simulink model "ardupilotsailboat"  (R2022b)
settings: Solver=VariableStepAuto  StartTime=0.0  StopTime=250  RelTol=1e-3
values from neighbouring files (symbols this model uses):
  Ixx = 1/120 * pi * rho * L * B * T * (4*T^2 + B^2)    (= 0.835683076278)    [parameterCalculations.m]
  m = 2    [parameterCalculations.m]
  m11 = m*k11    [parameterCalculations.m]
  m22 = m*k22    [parameterCalculations.m]
  Yv = Yv * (u^2)/(U^2)    (= -23.3298597446)    [parameterCalculations.m]
undefined symbols (not defined in the file or in its folder): Waypoints
libraries: cstblocks x6, simulink x1, vrlib x1
(part 1 of 2)
settings Model: Creator=ruben  LastModifiedBy=ruben
settings SolverCC: MaxConsecutiveZCs=10  MaxConsecutiveMinStep=9  ZeroCrossControl=DisableAll  ZeroCrossAlgorithm=Adaptive  SolverResetMethod=Robust
settings DebuggingCC: SignalInfNanChecking=warning  AlgebraicLoopMsg=error  ArtificialAlgebraicLoopMsg=error  BlockPriorityViolationMsg=error  MinStepSizeMsg=error  MaskedZcDiagnostic=error  IgnoredZcDiagnostic=none  MultiTaskCondExecSysMsg=warning  MultiTaskRateTransMsg=warning  CheckMatrixSingularityMsg=error  StateNameClashWarn=warning

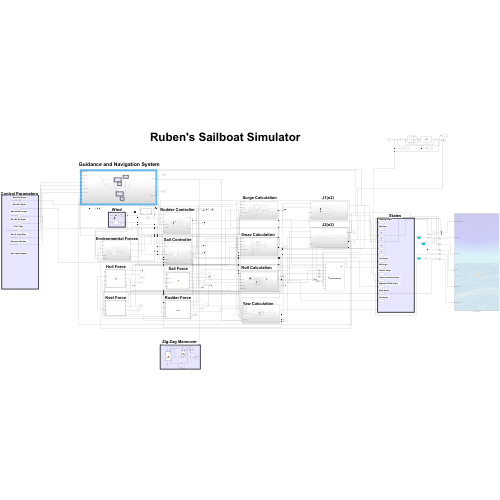
[thumbnail: Simulink's stored preview of the top-level diagram]
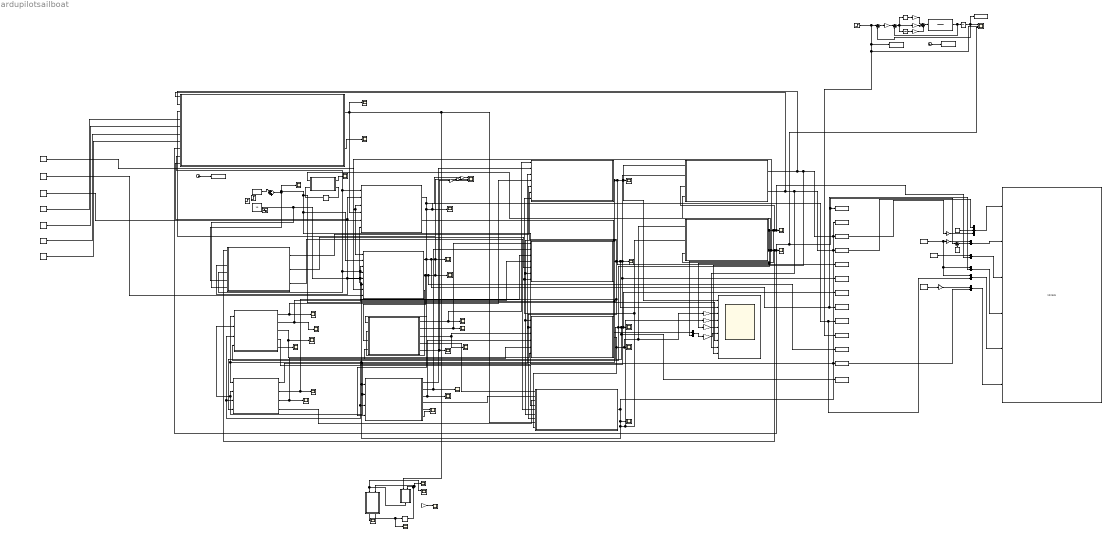
== system ardupilotsailboat ==
  note: Sail Force
  note: Ruben's Sailboat Simulator
  note: States
  note: x
  note: y
  note: Yaw Rate
  note: Heading Angle
  note: u
  note: v
  note: Roll Angle
  note: Sail Angle
  note: Rudder Angle
  note: Desired Heading Angle
  note: Apparent Wind Angle
  note: Wind Angle
  note: Roll Angle
  note: Guidance and Navigation System
  note: Environmental Forces
  note: Surge Calculation
  note: Sway Calculation
  note: Roll Calculation
  note: Yaw Calculation
  note: Wind
  note: Rudder Force
  note: Keel Force
  note: Hull Force
  note: Sail Controller
  note: Rudder Controller
  note: Zig-Zag Maneuver
  note: Control Parameters
  note: Max Sail Angle
  note: Min Sail Angle
  note: Sail No Go Angle
  note: Sail X-Track Max
  note: Sail Loiter Raduis
  note: Waypoint Radius
  note: Tack Type
  note: Max Rudder Angle
  note: J1(n2)
  note: J2(n2)
  Bus Creator : BusCreator  Inputs=2
  Clock : Clock
  Clock2 : Clock
  Cross-Track Distance(m) : Constant  Value=7.5
  Delay1 : Delay  DelayLength=1  SampleTime=0.01
  Delay2 : Delay  DelayLength=1  SampleTime=0.01
  Derivative : Derivative
  Gain : Gain  Gain=0.0225
  Gain{1..8} (8 alike) : Gain  Gain=180/pi
  Gain10 : Gain
  Gain11 : Gain  Gain=0.99
  Gain9 : Gain  Gain=2.66
  Integrator : Integrator
  Integrator1 : Integrator
  MATLAB Function1 : MATLAB Function  TreatAsAtomicUnit=on
  MATLAB Function3 : MATLAB Function  TreatAsAtomicUnit=on
  MATLAB Function4 : MATLAB Function  TreatAsAtomicUnit=on
  MATLAB Function5 : MATLAB Function  TreatAsAtomicUnit=on
  MATLAB Function6 : MATLAB Function  TreatAsAtomicUnit=on
  MATLAB Function7 : MATLAB Function  TreatAsAtomicUnit=on
  MATLAB Function8 : MATLAB Function  TreatAsAtomicUnit=on
  Mux1 : Mux  Inputs=3
  Mux{2,4..7} (5 alike) : Mux  Inputs=2
  Radius of Acceptance(m) : Constant  Value=5
  Roll Axis of Rotation : Constant  Value=[ -1 0 0 ]
  Scope{,1..14,16..17,33,35,37..38,40,42} (23 alike) : Scope
  Scope15 : Scope  NumInputPorts=3
  Scope18 : Scope  NumInputPorts=3
  Scope36 : Scope  NumInputPorts=9
  Scope41 : Scope  NumInputPorts=2
  Sine Wave : Sin  Amplitude=0.1  Frequency=0.1  SampleTime=0
  Step : Step  Time=19  After=0.25  SampleTime=0
  Step1 : Step  Time=40  After=0.5  SampleTime=0
  Step2 : Step  After=0.1  SampleTime=0
  Subsystem1 : Subsystem
  Subsystem10 : Subsystem
  Subsystem2 : Subsystem
  Subsystem3 : Subsystem
  Subsystem4 : Subsystem
  Subsystem5 : Subsystem
  Subsystem6 : Subsystem
  Subsystem7 : Subsystem
  Subsystem8 : Subsystem
  Subsystem9 : Subsystem
  Sum : Sum  Inputs=|++-+
  Sum1 : Sum  Inputs=|+-  SaturateOnIntegerOverflow=on
  Sum2 : Sum  Inputs=|+-
  Sum3 : Sum  Inputs=|+++
  Sum4 : Sum  Inputs=|+-
  "Tack Type (1:Direct, 2:Indirect 3:Zone)" : Constant
  To Workspace : ToWorkspace  VariableName=yawrate  SaveFormat=Timeseries  SampleTime=-1
  To Workspace1 : ToWorkspace  VariableName=yaw  SaveFormat=Timeseries  SampleTime=-1
  To Workspace10 : ToWorkspace  VariableName=psid  SaveFormat=Timeseries  SampleTime=-1
  To Workspace11 : ToWorkspace  VariableName=awa  SaveFormat=Timeseries  SampleTime=-1
  To Workspace12 : ToWorkspace  VariableName=wind  SaveFormat=Timeseries  SampleTime=-1
  To Workspace13 : ToWorkspace  VariableName=roll  SaveFormat=Timeseries  SampleTime=-1
  To Workspace14 : ToWorkspace  VariableName=time1  SaveFormat=Timeseries  SampleTime=-1
  To Workspace15 : ToWorkspace  VariableName=time  SaveFormat=Timeseries  SampleTime=-1
  To Workspace16 : ToWorkspace  VariableName=step  SaveFormat=Timeseries  SampleTime=-1
  To Workspace2 : ToWorkspace  VariableName=simout  SaveFormat=Timeseries  SampleTime=-1
  To Workspace3 : ToWorkspace  VariableName=x  SaveFormat=Timeseries  SampleTime=-1
  To Workspace4 : ToWorkspace  VariableName=y  SaveFormat=Timeseries  SampleTime=-1
  To Workspace5 : ToWorkspace  VariableName=u  SaveFormat=Timeseries  SampleTime=-1
  To Workspace6 : ToWorkspace  VariableName=v  SaveFormat=Timeseries  SampleTime=-1
  To Workspace7 : ToWorkspace  VariableName=phi  SaveFormat=Timeseries  SampleTime=-1
  To Workspace8 : ToWorkspace  VariableName=delta_s  SaveFormat=Timeseries  SampleTime=-1
  To Workspace9 : ToWorkspace  VariableName=delta_r  SaveFormat=Timeseries  SampleTime=-1
  Transfer Fcn : TransferFcn  Numerator=[2.5]  Denominator=[0.4 1 ]
  VR Sailing Yacht Animation : vrlib/VR Sink  InstantiateOnLoad=on  SampleTime=0.05  ViewEnable=on  RemoteChange=off  RemoteView=off  FieldsWritten=Hull_EarthFixed.translation.3.1.1.double#Rot_Yaw.rotation.4.1.1.double#Rot_Roll.rotation.4.1.1.double#Sail.rotation.4.1.1.double#Rudder.rotation.4.1.1.double#Wind_Arrow.rotation.4.1.1.double  WorldFileName=SailingYachtAnimation.wrl  WorldDescription=Sailing Yacht VR animation  AutoView=on  VideoDimensions=[]  AllowVariableSize=off  FigureProperties="{'Position', 'Name', 'Viewpoint', 'CameraBound', 'CameraDirection', 'CameraPosition', 'CameraUpVector', 'ZoomFactor', 'Antialiasing', 'Headlight', 'Lighting', 'NavPanel', 'Sound', 'StatusBar', 'Stereo3D', 'Stereo3DCameraOffset', 'Stereo3DHIT', 'ToolBar', 'Textures', 'Transparency', 'Triad', 'Wireframe', 'NavZones', 'NavMode', 'NavSpeed', 'CaptureFileFormat', 'CaptureFileName', 'Record2DCompressMethod', 'Record2DCompressQuality', 'Record2D', 'Record2DFileName', 'Record2DFPS'; [9.6200000000000000e+02   8.4000000000000000e+01   9.5800000000000000e+02   3.8020000000000005e+02], 'Sailing Yacht VR animation', 'North', 'on', [0.0000000000000000e+00   0.0000000000000000e+00  -1.0000000000000000e+00], [0.0000000000000000e+00   0.0000000000000000e+00   2.5000000000000000e+01], [0.0000000000000000e+00   1.0000000000000000e+00   0.0000000000000000e+00], [1.0000000000000000e+00], 'off', 'on', 'on', 'halfbar', 'on', 'on', 'off', [1.0000000149011612e-01], [0.0000000000000000e+00], 'on', 'on', 'on', 'none', 'off', 'off', 'fly', 'veryfast', 'tif', '%f_anim_%n.tif', 'auto', [7.5000000000000000e+01], 'off', '%f_anim_%n.avi', 'auto'}"
  Yaw Axis of Rotation : Constant  Value=[ 0 1 0 ]
  Yaw Axis of Rotation1 : Constant  Value=[ 0 1 0 ]
  apparent wind : Scope
  max rudder angle(Rad) : Constant  Value=pi/6
  max sail angle(Rad) : Constant  Value=pi/3
  min sail angle(Rad) : Constant  Value=-pi/3
  rudder and psi1 : Scope  NumInputPorts=2
  rudder angle5 : Scope
  rudder angle6 : Scope
  rudder angle7 : Scope  NumInputPorts=3
  rudder angle8 : Scope
  rudder_angle1 : Scope
  sail angle : Scope
  sail no go angle(Degrees) : Constant  Value=45
  wind direction : Constant  Value=pi/2
  wind velocity : Constant  Value=10
  z : Constant  Value=0
  z - y1 : Gain  Gain=-1
  z - y2 : Gain  Gain=-1
  z - y3 : Gain  Gain=-1
  z1 : Constant  Value=pi/2
  wires:
  Subsystem1/2(heading (degrees)) -> Scope33/1
  MATLAB Function3/2(Ys) -> Scope1/1, Subsystem4/1(sail force (Ys))
  MATLAB Function3/3(Ks) -> Scope14/1, Subsystem5/3(sail force (Ks))
  MATLAB Function3/4(Ns) -> Subsystem6/1(sail force (Ns))
  MATLAB Function4/1(Xr) -> Subsystem2/2(rudder force (Xr))
  MATLAB Function4/2(Yr) -> Scope2/1, Subsystem4/2(rudder force (Yr))
  MATLAB Function4/3(Kr) -> Scope13/1, Subsystem5/4(hull force(Kh))
  MATLAB Function4/4(Nr) -> Subsystem6/2(rudder force (Nr))
  MATLAB Function5/1(Xk) -> Subsystem2/3(keel force (Xk))
  MATLAB Function5/2(Yk) -> Scope3/1, Subsystem4/3(keel force (Yk))
  MATLAB Function5/3(Kk) -> Scope12/1, Subsystem5/5(keel force (Kk))
  MATLAB Function5/4(Nk) -> Subsystem6/3(keel force (Nk))
  MATLAB Function6/1(Xh) -> Scope5/1, Subsystem2/4(hull force (Xh))
  MATLAB Function6/3(Kh) -> Scope11/1, Subsystem5/6(rudder force (Kr))
  MATLAB Function6/4(Nh) -> Subsystem6/4(hull force (Nh))
  Subsystem4/1(v) -> Scope36/2, Scope8/1, Subsystem9/2(v), To Workspace6/1, MATLAB Function6/3(v), MATLAB Function5/3(v), MATLAB Function4/3(v), Subsystem2/6(v), Subsystem6/7(v), Subsystem5/2(v), Subsystem8/2(v), Subsystem1/10(v), Subsystem3/3(v), Subsystem7/4(v)
  Subsystem3/1(Xe) -> Subsystem2/5(environmental force (Xe))
  Subsystem3/2(Ye) -> Subsystem4/5(environmental force (Ye))
  Subsystem3/3(Ne) -> Subsystem6/5(environmental force (Ne))
  Subsystem2/1(u) -> MATLAB Function5/2(u), MATLAB Function6/2(u), MATLAB Function4/2(u), Subsystem1/9(u), Subsystem8/1(u), Subsystem3/4(u), Subsystem7/3(u), Subsystem6/6(u), Subsystem5/1(u), Subsystem4/6(u), To Workspace5/1, Scope36/1, Subsystem9/1(u), Scope35/1
  Subsystem6/1(r) -> Subsystem8/6(r), Subsystem7/6(r), MATLAB Function5/1(r), MATLAB Function6/1(r), MATLAB Function4/1(r), Gain4/1, Subsystem10/2(r), Subsystem2/7(r), Subsystem4/7(r), Scope40/1, To Workspace/1
  Subsystem5/1(p) -> Subsystem6/9(p), Subsystem10/1(p), Gain5/1, Scope38/1
  Subsystem10/1(Phi) -> Gain3/1, MATLAB Function5/4(phi), MATLAB Function6/4(phi), To Workspace13/1, MATLAB Function3/4(phi), To Workspace7/1, Scope37/1, Subsystem10/3(phi), Subsystem9/3(phi), Mux6/2, Scope9/1
  Clock2/1 -> To Workspace14/1
  MATLAB Function7/2(nextState) -> rudder angle5/1, Delay1/1
  Delay1/1 -> rudder angle8/1, MATLAB Function8/2(state), MATLAB Function7/2(currentState)
  MATLAB Function7/1(y) -> rudder angle6/1
  MATLAB Function8/1(y) -> MATLAB Function7/1(r), rudder angle7/1
  Gain2/1 -> rudder and psi1/1
  wind velocity/1 -> Subsystem3/6(wind Velocity), Subsystem7/5(wind velocity)
  Subsystem7/1(sail angle) -> MATLAB Function3/1(delta_s), Gain7/1, sail angle/1, Mux5/2, To Workspace8/1
  Subsystem7/2(alpha_aw) -> To Workspace11/1, Subsystem1/3(wind Direction), apparent wind/1, MATLAB Function3/3(apparent_wind_angle)
  Subsystem7/3(V_aw) -> MATLAB Function3/2(apparent_velocity)
  Subsystem8/1(rudder angle) -> Gain8/1, To Workspace9/1, Mux7/2, rudder_angle1/1, MATLAB Function4/4("delta_r ")
  MATLAB Function4/5(delta_r) -> Scope41/1
  MATLAB Function4/6(alpha_a) -> Scope41/2
  MATLAB Function6/2(Yh) -> Subsystem4/4(hull force (Yh)), Scope4/1
  max sail angle(Rad)/1 -> Subsystem7/7(max sail angle)
  min sail angle(Rad)/1 -> Subsystem7/8(min sail angle)
  max rudder angle(Rad)/1 -> Subsystem8/5(max rudder angle)
  sail no go angle(Degrees)/1 -> Subsystem1/4(no go Angle)
  "Tack Type (1:Direct, 2:Indirect 3:Zone)"/1 -> Subsystem1/5(tack Type)
  Cross-Track Distance(m)/1 -> Subsystem1/6(Cross-Track Distance)
  Radius of Acceptance(m)/1 -> Subsystem1/7(radius of acceptance)
  wind direction/1 -> Sum/1
  MATLAB Function6/5(Frh) -> Scope6/1
  MATLAB Function3/1(Xs) -> Subsystem2/1(sail force (Xs)), Scope7/1
  Subsystem9/2(y) -> Subsystem1/1(x position of Sailboat), Scope36/8, Mux1/1, To Workspace3/1
  Subsystem8/2(rudder angle1) -> Bus Creator/1
  Subsystem10/2(Psi) -> MATLAB Function1/1(psi), Bus Creator/2, Subsystem9/4(psi), Subsystem7/1(psi), Subsystem8/3(psi), Subsystem3/1(psi), Scope18/3, Sum1/1, To Workspace1/1, Subsystem1/8(psi), Scope10/1
  Bus Creator/1 -> Gain1/1
  z1/1 -> Sum1/2
  z - y1/1 -> Mux4/1
  Yaw Axis of Rotation/1 -> Mux5/1, Mux7/1, z - y1/1
  z/1 -> Mux1/2
  z - y3/1 -> Mux2/1
  Mux2/1 -> VR Sailing Yacht Animation/6
  Sum1/1 -> Mux4/2
  Yaw Axis of Rotation1/1 -> z - y3/1
  z - y2/1 -> Mux1/3
  Roll Axis of Rotation/1 -> Mux6/1
  Mux1/1 -> VR Sailing Yacht Animation/1
  Mux4/1 -> VR Sailing Yacht Animation/2
  Mux6/1 -> VR Sailing Yacht Animation/3
  Mux5/1 -> VR Sailing Yacht Animation/4
  Mux7/1 -> VR Sailing Yacht Animation/5
  Subsystem9/1(x) -> Subsystem1/2(y position of Sailboat), Scope36/9, z - y2/1, To Workspace4/1
  MATLAB Function3/5(awa) -> Gain6/1, Scope42/1
  Gain3/1 -> Scope36/5
  Gain1/1 -> Scope36/6
  Gain4/1 -> Scope36/4
  Gain5/1 -> Scope36/3
  Gain6/1 -> Scope15/3
  Gain7/1 -> Scope15/2
  Gain8/1 -> Scope15/1
  MATLAB Function1/2(nextState) -> Delay2/1
  Delay2/1 -> MATLAB Function1/2(currentState)
  MATLAB Function1/1(y) -> Scope16/1
  Sum/1 -> Scope17/1, Scope36/7, Mux2/2, To Workspace12/1, Subsystem7/2(wind direction), Subsystem3/5(wind Direction)
  Clock/1 -> To Workspace15/1
  Integrator/1 -> Gain10/1
  Derivative/1 -> Gain/1
  Gain9/1 -> Sum3/2
  Transfer Fcn/1 -> Sum2/2, Integrator1/1
  Sum2/1 -> Derivative/1, Gain9/1, Integrator/1
  Gain/1 -> Sum3/1
  Sum3/1 -> Transfer Fcn/1
  Gain10/1 -> Sum3/3
  Step2/1 -> Sum4/1, Scope18/2, To Workspace10/1, To Workspace16/1
  Integrator1/1 -> Sum4/2, Scope18/1, To Workspace2/1
  Sum4/1 -> Gain11/1
  Gain11/1 -> Sum2/1
  Subsystem1/1(heading (rad)) -> Scope/1, Subsystem8/4(desired heading), Subsystem6/8(desired heading), MATLAB Function8/1(psi)

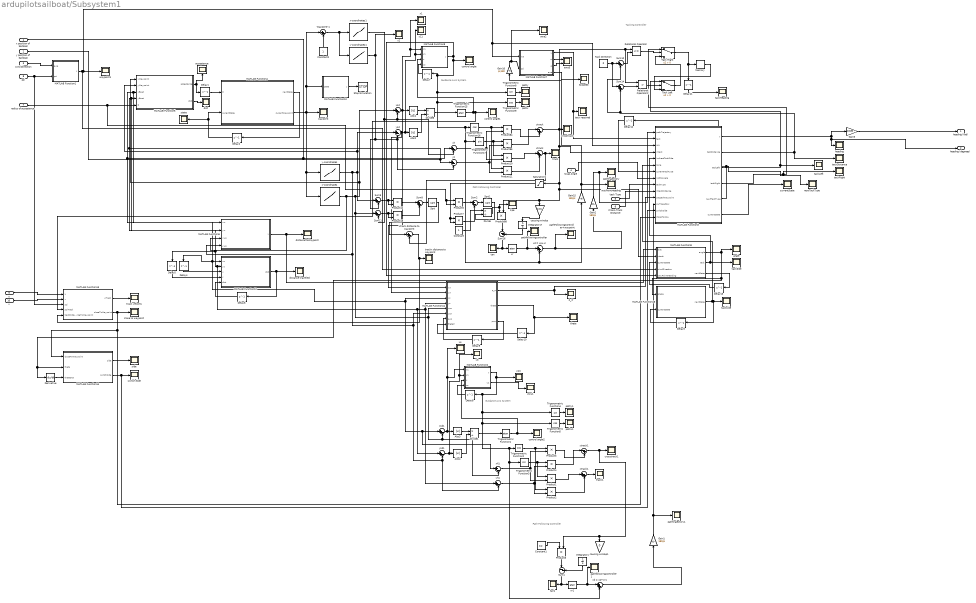
== system ardupilotsailboat/Subsystem1 ==
  note: Guidance Axis System
  note: Tacking Controller
  note: Path Following Controller
  note: Guidance Axis System
  note: Path Following Controller
  x position of Sailboat : Inport
  y position of Sailboat : Inport  Port=2
  wind Direction : Inport  Port=3
  no go Angle : Inport  Port=4
  tack Type : Inport  Port=5
  Cross-Track Distance : Inport  Port=6
  radius of acceptance : Inport  Port=7
  psi : Inport  Port=8
  u : Inport  Port=9
  v : Inport  Port=10
  Abs{1..4} (4 alike) : Abs  SaturateOnIntegerOverflow=off
  Constant : Constant
  Constant1 : Constant  Value=0.2
  Constant2 : Constant
  Delay{1..2,4..12} (11 alike) : Delay  DelayLength=1
  Delay13 : Delay  DelayLength=1  SampleTime=2
  Delay3 : Delay  DelayLength=1  SampleTime=2
  Derivative : Derivative
  Divide : Product  Inputs=*/
  Divide1 : Product  Inputs=*/
  Divide6 : Product  Inputs=*/
  Gain1 : Gain  Gain=180/pi
  Gain10 : Gain  Gain=pi/180
  Gain15 : Gain  Gain=180/pi
  Gain2 : Gain  Gain=180/pi
  Gain3 : Gain  Gain=pi/180
  Integrator1 : Integrator  LimitOutput=on  UpperSaturationLimit=10  LowerSaturationLimit=-10
  Integrator17 : Integrator  LimitOutput=on  UpperSaturationLimit=pi/10  LowerSaturationLimit=-pi/10
  Kpe : Scope
  MATLAB Function1 : MATLAB Function  TreatAsAtomicUnit=on
  MATLAB Function10 : MATLAB Function  TreatAsAtomicUnit=on
  MATLAB Function11 : MATLAB Function  TreatAsAtomicUnit=on
  MATLAB Function12 : MATLAB Function  TreatAsAtomicUnit=on
  MATLAB Function13 : MATLAB Function  TreatAsAtomicUnit=on
  MATLAB Function14 : MATLAB Function  TreatAsAtomicUnit=on
  MATLAB Function18 : MATLAB Function  TreatAsAtomicUnit=on
  MATLAB Function2 : MATLAB Function  TreatAsAtomicUnit=on
  MATLAB Function3 : MATLAB Function  TreatAsAtomicUnit=on
  MATLAB Function4 : MATLAB Function  TreatAsAtomicUnit=on
  MATLAB Function5 : MATLAB Function  TreatAsAtomicUnit=on
  MATLAB Function6 : MATLAB Function  TreatAsAtomicUnit=on
  MATLAB Function7 : MATLAB Function  TreatAsAtomicUnit=on
  MATLAB Function8 : MATLAB Function  TreatAsAtomicUnit=on
  MATLAB Function9 : MATLAB Function  TreatAsAtomicUnit=on
  Memory : Memory
  Product{1..7,10..13,84..85,88} (14 alike) : Product
  Relational Operator : RelationalOperator  Operator=<=  OutDataTypeStr=boolean  RndMeth=Simplest  InputSameDT=off
  Relational Operator1 : RelationalOperator  Operator=>  OutDataTypeStr=boolean  RndMeth=Simplest  InputSameDT=off
  Saturation1 : Saturate  UpperLimit=4.9  LowerLimit=-4.9
  Scope33 : Scope
  Sqrt : Sqrt
  Sqrt1 : Sqrt
  Stop Simulation : Stop
  Sum1 : Sum  Inputs=|--
  Sum{2,9..11} (4 alike) : Sum  Inputs=|+-
  Sum14 : Sum  Inputs=|++
  Sum16 : Sum  Inputs=|--
  Sum8 : Sum  Inputs=|++
  Tack Direction : Constant  Value=0
  Tack Left : Switch  Criteria=u2 > Threshold  SaturateOnIntegerOverflow=off  InputSameDT=off
  Tack Right : Switch  Criteria=u2 > Threshold  SaturateOnIntegerOverflow=off  InputSameDT=off
  Trigonometric Function1 : Trigonometry  Operator=atan
  Trigonometric Function15 : Trigonometry  Operator=atan
  Trigonometric Function{2,5,9,16} (4 alike) : Trigonometry  Operator=cos
  Trigonometric Function{3..4,8,17} (4 alike) : Trigonometry
  Waypoint-1 : Sum  Inputs=|+-
  acceptance : Scope
  angle : Scope
  awa2 : Scope
  awa3 : Scope  NumInputPorts=2
  causing windup : Gain  Gain=0.01
  causing windup1 : Gain  Gain=0
  close to waypoint : Scope
  control angle : Scope
  control angle1 : Scope
  control angle2 : Scope
  crosstrack : Scope
  crosstrack1 : Scope
  currentState : Scope
  dist : Scope
  distance travelled : Scope
  distanceToWaypoint : Scope
  heading : Scope
  nextTackType : Scope
  p_w : Scope
  "pathFollowingController+waypoint " : Scope
  pathfollowingcontroller : Scope
  pathfollowingcontroller1 : Scope
  pathtrajectory : Scope
  pathtrajectory1 : Scope
  pathx : Scope
  pathx1 : Scope
  pathy : Scope
  pathy1 : Scope
  pwu1 : Scope
  side : Scope
  state : Scope
  switch Side : Scope
  tack required : Scope
  tackDistance : Scope
  tackHeading : Scope
  tackLeft : Scope
  tackRight : Scope
  tackSide : Scope
  tackside : Scope
  tan : Scope
  tan1 : Scope
  theta : Scope
  track : Scope
  track velocity : Scope
  track1 : Scope
  trackx distance to waypoint : Scope
  wayPointHeading : Scope
  waypoint : Scope
  waypoint1 : Scope
  x-coordinates : Lookup_n-D  NumberOfTableDimensions=1  BreakpointsForDimension1=Waypoints.number  Table=Waypoints.x  InterpMethod=Cubic spline  ExtrapMethod=Cubic spline  InternalRulePriority=Speed  RndMeth=Simplest
  x-coordinates1 : Lookup_n-D  NumberOfTableDimensions=1  BreakpointsForDimension1=Waypoints.number  Table=Waypoints.x  InterpMethod=Cubic spline  ExtrapMethod=Cubic spline  InternalRulePriority=Speed  RndMeth=Simplest
  x1 : Scope
  x2 : Scope
  x4 : Scope
  xd = xp+xr : Sum  Inputs=|++
  xd = xp+xr1 : Sum  Inputs=|++
  xh : Sum  Inputs=|+-
  xh1 : Sum  Inputs=|+-
  xr : Trigonometry  Operator=atan
  xr1 : Trigonometry  Operator=atan
  xsd : Sum  Inputs=|+-
  xsd1 : Sum  Inputs=|+-
  xtrack : Sum  Inputs=|++
  xtrack distance to waypoint : Sum  Inputs=|+-
  xtrack1 : Sum  Inputs=|++
  y-coordinates : Lookup_n-D  NumberOfTableDimensions=1  BreakpointsForDimension1=Waypoints.number  Table=Waypoints.y  InterpMethod=Cubic spline  ExtrapMethod=Cubic spline  InternalRulePriority=Speed  RndMeth=Simplest
  y-coordinates1 : Lookup_n-D  NumberOfTableDimensions=1  BreakpointsForDimension1=Waypoints.number  Table=Waypoints.y  InterpMethod=Cubic spline  ExtrapMethod=Cubic spline  InternalRulePriority=Speed  RndMeth=Simplest
  y11 : Scope
  y3 : Scope
  yh : Sum  Inputs=|+-
  yh1 : Sum  Inputs=|+-
  ypw : Scope
  ysd : Sum  Inputs=|+-
  ysd1 : Sum  Inputs=|+-
  ytrack : Sum  Inputs=|-+
  ytrack1 : Sum  Inputs=|-+
  heading (rad) : Outport
  heading (degrees) : Outport  Port=2
  wires:
  MATLAB Function11/2(theta) -> Delay10/1, theta/1
  MATLAB Function7/3(p) -> awa3/2
  Delay2/1 -> MATLAB Function4/2(currentState), state/1
  Trigonometric Function17/1 -> Product10/1, Product85/1
  MATLAB Function3/6(currentState) -> currentState/1
  MATLAB Function3/1(y) -> Gain3/1, heading (degrees)/1, heading/1
  Gain2/1 -> MATLAB Function3/1(pathTrajectory), pathtrajectory/1
  Delay12/1 -> MATLAB Function3/7(currentTackType)
  MATLAB Function4/2(currentWaypoint) -> MATLAB Function10/1(state), Waypoint-1/1, waypoint/1, x-coordinates/1, y-coordinates/1
  yh/1 -> Product85/2, Product11/2
  MATLAB Function7/2(w) -> awa3/1
  Sum14/1 -> Relational Operator1/2
  ytrack/1 -> Saturation1/1, Product88/2, causing windup/1, MATLAB Function9/2(xtrack), MATLAB Function3/4(xtrack), crosstrack/1, Relational Operator1/1, Relational Operator/1
  Product85/1 -> ytrack/1
  Delay11/1 -> tackHeading/1
  MATLAB Function3/2(tackDistance) -> Sum10/2, Sum14/2, tackDistance/1
  Integrator17/1 -> Sum16/2
  Abs1/1 -> Divide6/1
  Trigonometric Function16/1 -> Product11/1, Product84/1
  Delay7/1 -> MATLAB Function8/4(us)
  MATLAB Function18/1(nextState) -> tackside/1, Delay3/1, MATLAB Function3/6(zone)
  xd = xp+xr/1 -> "pathFollowingController+waypoint "/1, Gain2/1
  Gain10/1 -> MATLAB Function7/2(psi), awa2/1
  MATLAB Function3/5(nextTackType) -> Delay12/1, nextTackType/1
  Delay13/1 -> MATLAB Function9/3(currentState)
  Waypoint-1/1 -> x-coordinates1/1, y-coordinates1/1
  Delay3/1 -> MATLAB Function18/2(currentState)
  xsd/1 -> MATLAB Function11/1(xw), MATLAB Function8/1(x1), x1/1, Abs1/1
  Constant2/1 -> Waypoint-1/2
  MATLAB Function8/1(y) -> Trigonometric Function8/1, Trigonometric Function9/1, Trigonometric Function17/1, xd = xp+xr/2, Gain15/1, Trigonometric Function16/1, Delay7/1, control angle/1, MATLAB Function9/5(wayPointHeading)
  xh/1 -> Product84/2, Product10/2
  Delay1/1 -> MATLAB Function4/1(R)
  MATLAB Function9/3(nextState) -> Delay13/1
  Product84/1 -> ytrack/2
  y-coordinates1/1 -> yh/2, ysd/2, Sum9/2, x2/1
  Trigonometric Function15/1 -> MATLAB Function13/4(psiTrack), control angle1/1, MATLAB Function8/3(u)
  ysd/1 -> y11/1, MATLAB Function8/2(y1), Abs2/1, MATLAB Function11/2(yw)
  x-coordinates1/1 -> Sum11/2, xh/2, xsd/2
  Sum16/1 -> xr/1, tan/1
  Product13/1 -> Sum8/2
  Gain15/1 -> Gain10/1, wayPointHeading/1
  MATLAB Function6/1(y) -> MATLAB Function9/1(dist), distanceToWaypoint/1
  Delay5/1 -> MATLAB Function12/4(y)
  MATLAB Function9/1(angle) -> angle/1, Derivative/1, MATLAB Function14/2(theta), MATLAB Function18/1(angle)
  Product88/1 -> Sum16/1
  Relational Operator1/1 -> Tack Left/2
  MATLAB Function3/3(tackLeft) -> Tack Left/1, tackLeft/1
  Tack Right/1 -> Memory/1, Delay11/1
  xtrack distance to waypoint/1 -> MATLAB Function13/5(trackDistanceToWaypoint), trackx distance to waypoint/1
  Memory/1 -> Tack Left/3
  Product11/1 -> xtrack/2
  Trigonometric Function8/1 -> pathy/1
  MATLAB Function7/1(y) -> MATLAB Function3/2(tack), tack required/1
  Delay4/1 -> MATLAB Function12/3(x)
  causing windup/1 -> Integrator17/1
  Tack Left/1 -> Tack Right/3
  MATLAB Function10/1(y) -> Stop Simulation/1
  Sum8/1 -> Sqrt/1
  Sum11/1 -> Product13/2, Product13/1
  Tack Direction/1 -> Sum14/1, Sum10/1
  Sum9/1 -> Product12/1, Product12/2
  Delay6/1 -> MATLAB Function12/5("dist ")
  MATLAB Function5/1(acceptance) -> Delay1/1, acceptance/1
  MATLAB Function12/1(dist) -> distance travelled/1, Delay6/1
  Relational Operator/1 -> Tack Right/2
  Sum10/1 -> Relational Operator/2
  xtrack/1 -> xtrack distance to waypoint/2, track/1
  Abs2/1 -> Divide6/2
  MATLAB Function4/1(nextState) -> Delay2/1
  Sqrt/1 -> xtrack distance to waypoint/1
  MATLAB Function11/1(p_w) -> p_w/1, MATLAB Function3/11(passedWaypoint)
  Product10/1 -> xtrack/1
  xr/1 -> xd = xp+xr/1, pathfollowingcontroller/1
  MATLAB Function3/4(tackRight) -> tackRight/1, Tack Right/1
  Product12/1 -> Sum8/1
  Trigonometric Function9/1 -> pathx/1
  MATLAB Function7/4(awa) -> Scope33/1
  no go Angle/1 -> MATLAB Function3/8(noGoAngle)
  tack Type/1 -> MATLAB Function3/9(tackType)
  Cross-Track Distance/1 -> MATLAB Function3/10(XtrackDistance)
  radius of acceptance/1 -> Product6/2, Product6/1, MATLAB Function5/5(R)
  MATLAB Function9/2(tack) -> MATLAB Function3/5(indirectTackSide), tackSide/1
  MATLAB Function5/2(dist) -> dist/1
  wind Direction/1 -> MATLAB Function1/1(awa)
  psi/1 -> MATLAB Function13/3(psi), MATLAB Function1/2(psi)
  MATLAB Function1/1(y) -> waypoint1/1, MATLAB Function7/1(wa), MATLAB Function3/3(WA), MATLAB Function9/4(windDirection)
  Divide6/1 -> Trigonometric Function15/1
  Divide1/1 -> Trigonometric Function1/1
  Product2/1 -> xtrack1/2
  Trigonometric Function5/1 -> pathx1/1
  Product1/1 -> xtrack1/1
  Abs4/1 -> Divide1/2
  Trigonometric Function4/1 -> pathy1/1
  y-coordinates/1 -> yh1/2, ysd1/2, MATLAB Function11/6(ycw), MATLAB Function6/4(ywp), MATLAB Function5/2(yWaypoint), ysd/1, Sum9/1
  xtrack1/1 -> track1/1
  xh1/1 -> Product3/2, Product1/2
  Abs3/1 -> Divide1/1
  ysd1/1 -> y3/1, MATLAB Function2/2(y1), Abs4/1
  x-coordinates/1 -> MATLAB Function6/3(xwp), xh1/2, xsd1/2, MATLAB Function11/5(xcw), Sum11/1, xsd/1, MATLAB Function5/1(xWaypoint)
  Product3/1 -> ytrack1/2
  Trigonometric Function2/1 -> Product2/1, Product3/1
  Product4/1 -> ytrack1/1
  Trigonometric Function3/1 -> Product1/1, Product4/1
  yh1/1 -> Product4/2, Product2/2
  xsd1/1 -> x4/1, MATLAB Function2/1(x1), Abs3/1
  Trigonometric Function1/1 -> MATLAB Function2/3(u), control angle2/1
  Delay8/1 -> MATLAB Function2/4(us)
  xr1/1 -> xd = xp+xr1/1, pathfollowingcontroller1/1
  Product5/1 -> Sum1/1
  Constant1/1 -> Product5/1
  Sum1/1 -> xr1/1, tan1/1
  MATLAB Function2/1(y) -> ypw/1, Trigonometric Function4/1, Trigonometric Function5/1, xd = xp+xr1/2, Trigonometric Function3/1, Trigonometric Function2/1, Delay8/1
  xd = xp+xr1/1 -> Gain1/1
  Integrator1/1 -> Sum1/2
  ytrack1/1 -> Product5/2, causing windup1/1, crosstrack1/1
  Gain1/1 -> MATLAB Function3/12(pwTrajectory), pathtrajectory1/1
  MATLAB Function2/2(u1) -> pwu1/1
  x position of Sailboat/1 -> xh/1, xh1/1, xsd1/1, MATLAB Function11/3(xs), MATLAB Function12/1(xs), Delay4/1, MATLAB Function6/1(xw), MATLAB Function5/3(xBoat)
  y position of Sailboat/1 -> yh/1, MATLAB Function6/2(yw), MATLAB Function5/4(yBoat), ysd1/1, yh1/1, MATLAB Function11/4(ys), MATLAB Function12/2(ys), Delay5/1
  MATLAB Function11/3(pwn) -> Delay9/1
  Delay9/1 -> MATLAB Function11/7(pwc)
  Delay10/1 -> MATLAB Function11/8(thetaP)
  Sum2/1 -> Sqrt1/1
  Product6/1 -> Sum2/1
  Product7/1 -> Sum2/2
  Constant/1 -> Divide/1
  Sqrt1/1 -> Divide/2
  Divide/1 -> Product88/1, Kpe/1
  Saturation1/1 -> Product7/2, Product7/1
  Gain3/1 -> heading (rad)/1
  u/1 -> MATLAB Function13/1(u)
  v/1 -> MATLAB Function13/2(v)
  MATLAB Function13/1(uTrack) -> track velocity/1
  MATLAB Function13/2(closeToWaypoint) -> MATLAB Function3/14(closeToWay), MATLAB Function14/1(closeToWaypoint), close to waypoint/1
  Derivative/1 -> MATLAB Function14/3(thetaDot)
  MATLAB Function14/1(side) -> side/1
  MATLAB Function14/2(switchSide) -> MATLAB Function3/13(switchSide), switch Side/1

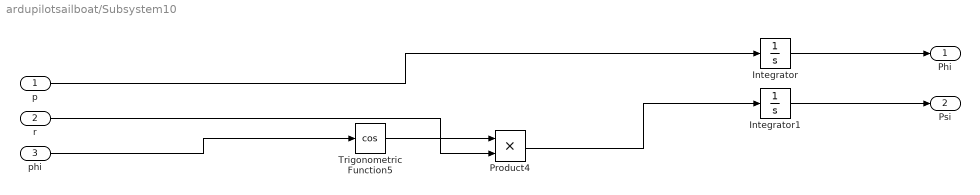
== system ardupilotsailboat/Subsystem10 ==
  p : Inport
  r : Inport  Port=2
  phi : Inport  Port=3
  Integrator : Integrator
  Integrator1 : Integrator
  Product4 : Product
  Trigonometric Function5 : Trigonometry  Operator=cos
  Phi : Outport
  Psi : Outport  Port=2
  wires:
  Integrator1/1 -> Psi/1
  Integrator/1 -> Phi/1
  p/1 -> Integrator/1
  Trigonometric Function5/1 -> Product4/1
  Product4/1 -> Integrator1/1
  r/1 -> Product4/2
  phi/1 -> Trigonometric Function5/1

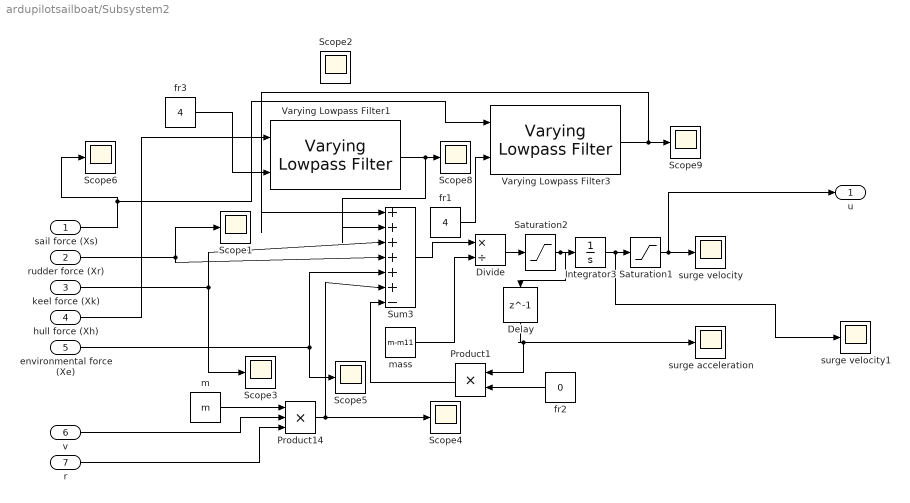
== system ardupilotsailboat/Subsystem2 ==
  sail force (Xs) : Inport
  rudder force (Xr) : Inport  Port=2
  keel force (Xk) : Inport  Port=3
  hull force (Xh) : Inport  Port=4
  environmental force (Xe) : Inport  Port=5
  v : Inport  Port=6
  r : Inport  Port=7
  Delay : Delay  DelayLength=1  InitialCondition=0
  Divide : Product  Inputs=*/
  Integrator3 : Integrator  InitialCondition=1  LimitOutput=on  UpperSaturationLimit=1.3  LowerSaturationLimit=-1.3
  Product1 : Product
  Product14 : Product  Inputs=3
  Saturation1 : Saturate  UpperLimit=1.3  LowerLimit=-1.3
  Saturation2 : Saturate  UpperLimit=0.01  LowerLimit=-0.01
  Scope{1..6,8..9} (8 alike) : Scope
  Sum3 : Sum  Inputs=|++++++-
  Varying Lowpass Filter1 : cstblocks/Linear Parameter Varying/Varying Lowpass Filter  N=1
  Varying Lowpass Filter3 : cstblocks/Linear Parameter Varying/Varying Lowpass Filter  N=1
  fr1 : Constant  Value=4
  fr2 : Constant  Value=0
  fr3 : Constant  Value=4
  m : Constant  Value=m
  mass : Constant  Value=m-m11
  surge acceleration : Scope
  surge velocity : Scope
  surge velocity1 : Scope
  u : Outport
  wires:
  Saturation1/1 -> u/1, surge velocity/1
  Integrator3/1 -> surge velocity1/1, Saturation1/1
  m/1 -> Product14/1
  Divide/1 -> Saturation2/1
  mass/1 -> Divide/2
  Sum3/1 -> Divide/1
  rudder force (Xr)/1 -> Scope1/1, Sum3/4
  keel force (Xk)/1 -> Scope3/1, Sum3/3
  environmental force (Xe)/1 -> Sum3/5, Scope5/1
  r/1 -> Product14/3
  fr3/1 -> Varying Lowpass Filter1/2
  Varying Lowpass Filter1/1 -> Sum3/2, Scope8/1
  sail force (Xs)/1 -> Varying Lowpass Filter3/1, Scope6/1
  v/1 -> Product14/2
  Varying Lowpass Filter3/1 -> Sum3/1, Scope9/1
  Product14/1 -> Sum3/6, Scope4/1
  fr1/1 -> Varying Lowpass Filter3/2
  hull force (Xh)/1 -> Varying Lowpass Filter1/1
  fr2/1 -> Product1/2
  Product1/1 -> Sum3/7
  Delay/1 -> Product1/1, surge acceleration/1
  Saturation2/1 -> Delay/1, Integrator3/1

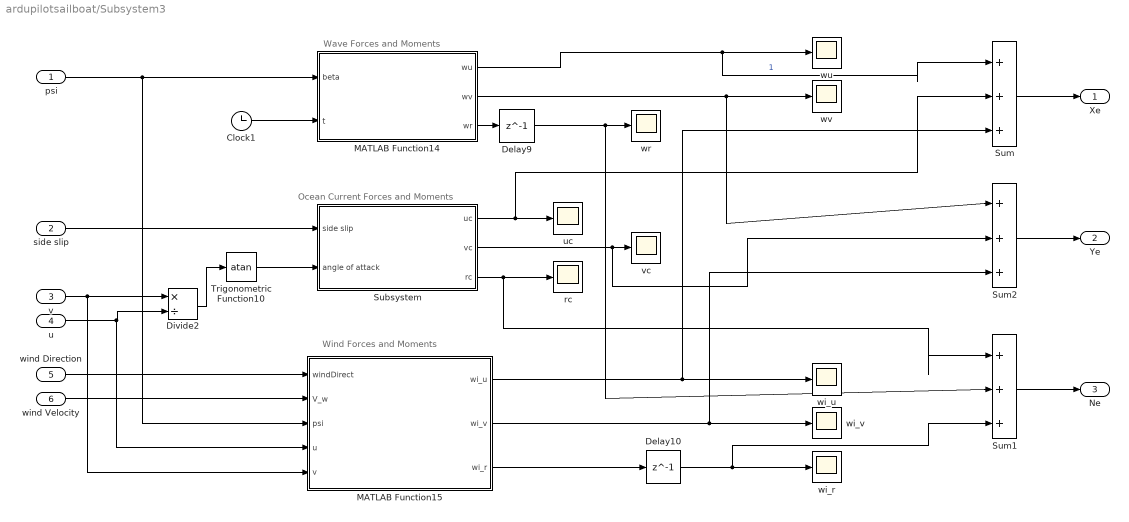
== system ardupilotsailboat/Subsystem3 ==
  note: Wave Forces and Moments
  note: Wind Forces and Moments
  note: Ocean Current Forces and Moments
  psi : Inport
  side slip : Inport  Port=2
  v : Inport  Port=3
  u : Inport  Port=4
  wind Direction : Inport  Port=5
  wind Velocity : Inport  Port=6
  Clock1 : Clock
  Delay10 : Delay  DelayLength=1
  Delay9 : Delay  DelayLength=1
  Divide2 : Product  Inputs=*/
  MATLAB Function14 : MATLAB Function  TreatAsAtomicUnit=on
  MATLAB Function15 : MATLAB Function  TreatAsAtomicUnit=on
  Subsystem : Subsystem
  Sum : Sum  Inputs=|+++
  Sum1 : Sum  Inputs=|+++
  Sum2 : Sum  Inputs=|+++
  Trigonometric Function10 : Trigonometry  Operator=atan
  rc : Scope
  uc : Scope
  vc : Scope
  wi_r : Scope
  wi_u : Scope
  wi_v : Scope
  wr : Scope
  wu : Scope
  wv : Scope
  Xe : Outport
  Ye : Outport  Port=2
  Ne : Outport  Port=3
  wires:
  MATLAB Function14/2(wv) -> Sum2/1, wv/1
  Trigonometric Function10/1 -> Subsystem/2(angle of attack)
  MATLAB Function14/3(wr) -> Delay9/1
  MATLAB Function15/2(wi_v) -> Sum2/3, wi_v/1
  Subsystem/1(uc) -> Sum/2, uc/1
  MATLAB Function15/3(wi_r) -> Delay10/1
  MATLAB Function15/1(wi_u) -> Sum/3, wi_u/1
  Clock1/1 -> MATLAB Function14/2(t)
  Subsystem/2(vc) -> Sum2/2, vc/1
  MATLAB Function14/1(wu) -> Sum/1, wu/1  "1"
  Divide2/1 -> Trigonometric Function10/1
  psi/1 -> MATLAB Function14/1(beta), MATLAB Function15/3(psi)
  side slip/1 -> Subsystem/1(side slip)
  v/1 -> MATLAB Function15/5(v), Divide2/1
  u/1 -> MATLAB Function15/4(u), Divide2/2
  wind Direction/1 -> MATLAB Function15/1(windDirect)
  wind Velocity/1 -> MATLAB Function15/2(V_w)
  Delay10/1 -> Sum1/3, wi_r/1
  Subsystem/3(rc) -> Sum1/1, rc/1
  Delay9/1 -> Sum1/2, wr/1
  Sum/1 -> Xe/1
  Sum2/1 -> Ye/1
  Sum1/1 -> Ne/1

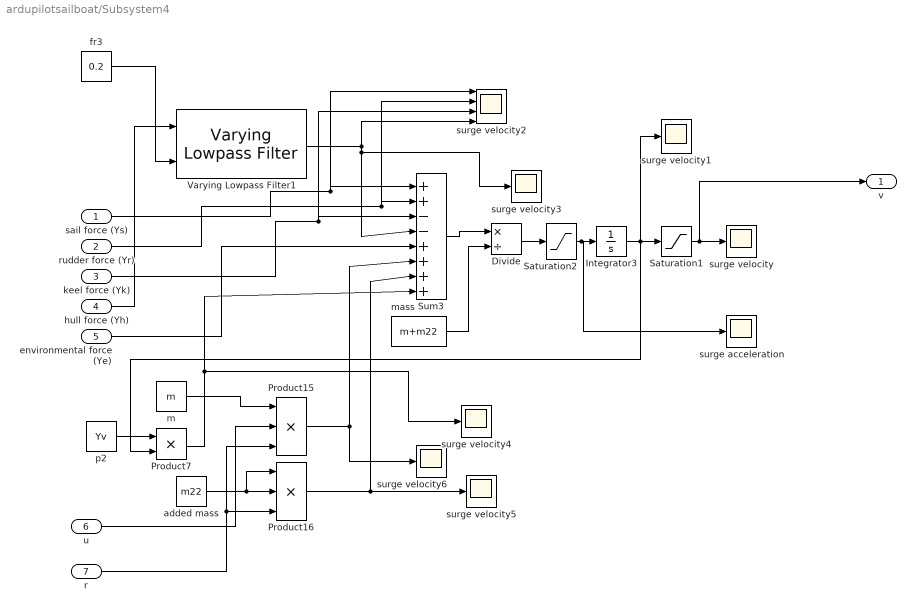
== system ardupilotsailboat/Subsystem4 ==
  sail force (Ys) : Inport
  rudder force (Yr) : Inport  Port=2
  keel force (Yk) : Inport  Port=3
  hull force (Yh) : Inport  Port=4
  environmental force (Ye) : Inport  Port=5
  u : Inport  Port=6
  r : Inport  Port=7
  Divide : Product  Inputs=*/
  Integrator3 : Integrator  UpperSaturationLimit=0.3  LowerSaturationLimit=-0.3
  Product15 : Product  Inputs=3
  Product16 : Product  Inputs=3
  Product7 : Product
  Saturation1 : Saturate  UpperLimit=0.3  LowerLimit=-0.3
  Saturation2 : Saturate  UpperLimit=0.05  LowerLimit=-0.05
  Sum3 : Sum  Inputs=|++--++++
  Varying Lowpass Filter1 : cstblocks/Linear Parameter Varying/Varying Lowpass Filter  N=1
  added mass : Constant  Value=m22
  fr3 : Constant  Value=0.2
  m : Constant  Value=m
  mass : Constant  Value=m+m22
  p2 : Constant  Value=Yv
  surge acceleration : Scope
  surge velocity{,1,3..6} (6 alike) : Scope
  surge velocity2 : Scope  NumInputPorts=4
  v : Outport
  wires:
  Integrator3/1 -> surge velocity1/1, Product7/2, Saturation1/1
  sail force (Ys)/1 -> surge velocity2/1, Sum3/1
  Divide/1 -> Saturation2/1
  mass/1 -> Divide/2
  Sum3/1 -> Divide/1
  rudder force (Yr)/1 -> surge velocity2/2, Sum3/2
  keel force (Yk)/1 -> surge velocity2/3, Sum3/3
  environmental force (Ye)/1 -> Sum3/5
  added mass/1 -> Product16/1, Product16/2
  p2/1 -> Product7/1
  m/1 -> Product15/1
  Product15/1 -> Sum3/6, surge velocity6/1
  Product16/1 -> Sum3/7, surge velocity5/1
  u/1 -> Product15/2
  r/1 -> Product16/3, Product15/3
  fr3/1 -> Varying Lowpass Filter1/2
  hull force (Yh)/1 -> Varying Lowpass Filter1/1
  Varying Lowpass Filter1/1 -> surge velocity3/1, Sum3/4, surge velocity2/4
  Saturation1/1 -> v/1, surge velocity/1
  Product7/1 -> surge velocity4/1, Sum3/8
  Saturation2/1 -> surge acceleration/1, Integrator3/1

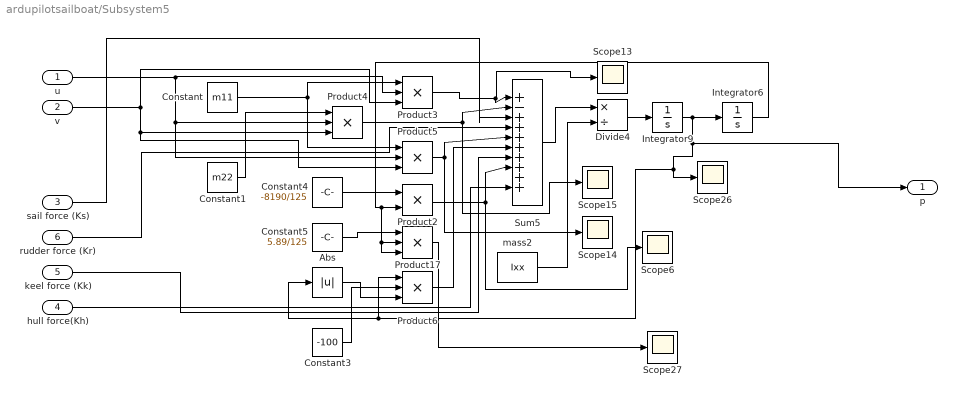
== system ardupilotsailboat/Subsystem5 ==
  u : Inport
  v : Inport  Port=2
  sail force (Ks) : Inport  Port=3
  hull force(Kh) : Inport  Port=4
  keel force (Kk) : Inport  Port=5
  rudder force (Kr) : Inport  Port=6
  Abs : Abs  SaturateOnIntegerOverflow=off
  Constant : Constant  Value=m11
  Constant1 : Constant  Value=m22
  Constant3 : Constant  Value=-100
  Constant4 : Constant  Value=-8190/125
  Constant5 : Constant  Value=5.89/125
  Divide4 : Product  Inputs=*/
  Integrator6 : Integrator
  Integrator9 : Integrator
  Product{3..6,17} (5 alike) : Product  Inputs=3
  Product2 : Product
  Scope{6,13..15,26..27} (6 alike) : Scope
  Sum5 : Sum  Inputs=|+-++++++++
  mass2 : Constant  Value=Ixx
  p : Outport
  wires:
  Product6/1 -> Sum5/6
  Abs/1 -> Product6/3
  Product4/1 -> Scope15/1, Sum5/2
  Constant3/1 -> Product6/2
  Integrator9/1 -> p/1, Abs/1, Product6/1, Scope26/1, Integrator6/1
  Integrator6/1 -> Product2/2, Product17/3, Product17/2
  Product17/1 -> Scope27/1
  Product2/1 -> Scope6/1, Sum5/8
  Constant/1 -> Product5/1, Product3/1
  Product3/1 -> Sum5/1, Scope13/1
  Constant5/1 -> Product17/1
  Product5/1 -> Scope14/1, Sum5/5
  Constant4/1 -> Product2/1
  Divide4/1 -> Integrator9/1
  mass2/1 -> Divide4/2
  Constant1/1 -> Product4/1
  Sum5/1 -> Divide4/1
  u/1 -> Product5/2, Product4/2, Product3/2
  v/1 -> Product3/3, Product5/3, Product4/3
  sail force (Ks)/1 -> Sum5/3
  rudder force (Kr)/1 -> Sum5/4
  hull force(Kh)/1 -> Sum5/10
  keel force (Kk)/1 -> Sum5/7

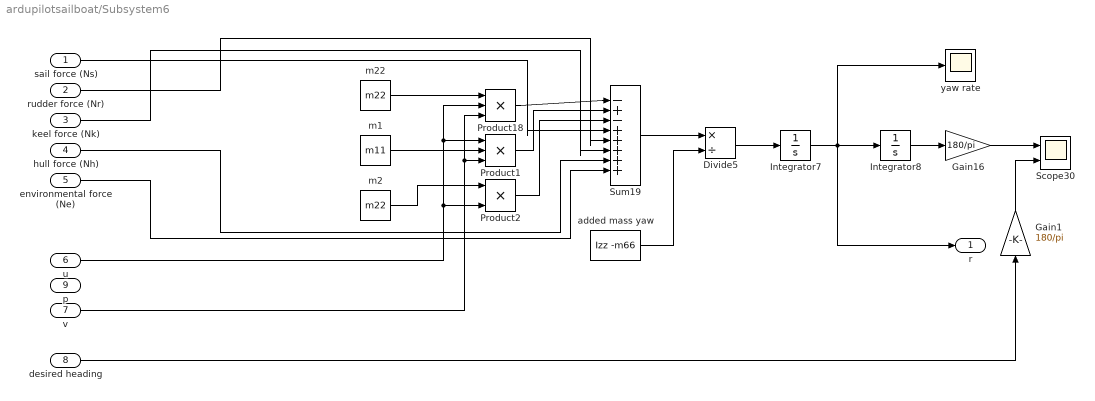
== system ardupilotsailboat/Subsystem6 ==
  sail force (Ns) : Inport
  rudder force (Nr) : Inport  Port=2
  keel force (Nk) : Inport  Port=3
  hull force (Nh) : Inport  Port=4
  environmental force (Ne) : Inport  Port=5
  u : Inport  Port=6
  v : Inport  Port=7
  desired heading : Inport  Port=8
  p : Inport  Port=9
  Divide5 : Product  Inputs=*/
  Gain1 : Gain  Gain=180/pi
  Gain16 : Gain  Gain=180/pi
  Integrator7 : Integrator
  Integrator8 : Integrator
  Product1 : Product  Inputs=3
  Product18 : Product  Inputs=3
  Product2 : Product  Inputs=3
  Scope30 : Scope  NumInputPorts=2
  Sum19 : Sum  Inputs=|-+-+++++
  added mass yaw : Constant  Value=Izz -m66
  m1 : Constant  Value=m11
  m2 : Constant  Value=m22
  m22 : Constant  Value=m22
  yaw rate : Scope
  r : Outport
  wires:
  Product18/1 -> Sum19/1
  Gain16/1 -> Scope30/1
  Product2/1 -> Sum19/3
  m22/1 -> Product18/1
  added mass yaw/1 -> Divide5/2
  m1/1 -> Product1/2
  Product1/1 -> Sum19/2
  Sum19/1 -> Divide5/1
  Integrator7/1 -> r/1, yaw rate/1, Integrator8/1
  Divide5/1 -> Integrator7/1
  sail force (Ns)/1 -> Sum19/4
  rudder force (Nr)/1 -> Sum19/5
  keel force (Nk)/1 -> Sum19/6
  hull force (Nh)/1 -> Sum19/7
  environmental force (Ne)/1 -> Sum19/8
  u/1 -> Product18/2, Product1/1, Product2/3
  v/1 -> Product1/3, Product18/3
  m2/1 -> Product2/1
  desired heading/1 -> Gain1/1
  Integrator8/1 -> Gain16/1
  Gain1/1 -> Scope30/2

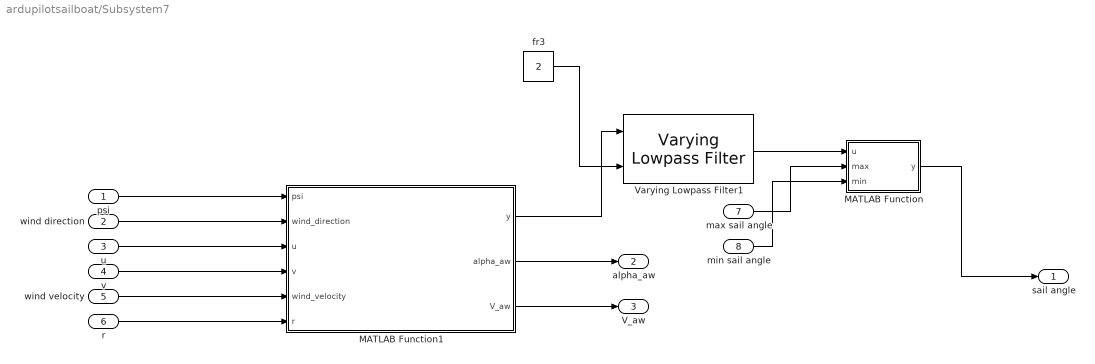
== system ardupilotsailboat/Subsystem7 ==
  psi : Inport
  wind direction : Inport  Port=2
  u : Inport  Port=3
  v : Inport  Port=4
  wind velocity : Inport  Port=5
  r : Inport  Port=6
  max sail angle : Inport  Port=7
  min sail angle : Inport  Port=8
  MATLAB Function : MATLAB Function  TreatAsAtomicUnit=on
  MATLAB Function1 : MATLAB Function  TreatAsAtomicUnit=on
  Varying Lowpass Filter1 : cstblocks/Linear Parameter Varying/Varying Lowpass Filter  N=1
  fr3 : Constant  Value=2
  sail angle : Outport
  alpha_aw : Outport  Port=2
  V_aw : Outport  Port=3
  wires:
  MATLAB Function1/1(y) -> Varying Lowpass Filter1/1
  fr3/1 -> Varying Lowpass Filter1/2
  r/1 -> MATLAB Function1/6(r)
  wind velocity/1 -> MATLAB Function1/5(wind_velocity)
  v/1 -> MATLAB Function1/4(v)
  u/1 -> MATLAB Function1/3(u)
  wind direction/1 -> MATLAB Function1/2(wind_direction)
  psi/1 -> MATLAB Function1/1(psi)
  MATLAB Function/1(y) -> sail angle/1
  MATLAB Function1/2(alpha_aw) -> alpha_aw/1
  MATLAB Function1/3(V_aw) -> V_aw/1
  Varying Lowpass Filter1/1 -> MATLAB Function/1(u)
  max sail angle/1 -> MATLAB Function/2(max)
  min sail angle/1 -> MATLAB Function/3(min)

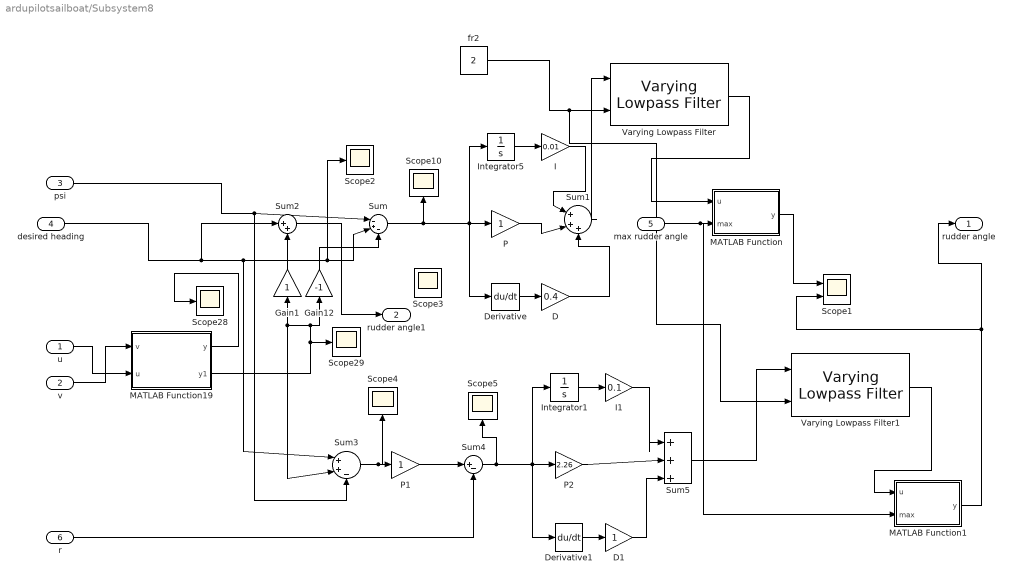
== system ardupilotsailboat/Subsystem8 ==
  u : Inport
  v : Inport  Port=2
  psi : Inport  Port=3
  desired heading : Inport  Port=4
  max rudder angle : Inport  Port=5
  r : Inport  Port=6
  D : Gain  Gain=0.4
  D1 : Gain
  Derivative : Derivative
  Derivative1 : Derivative
  Gain1 : Gain
  Gain12 : Gain  Gain=-1
  I : Gain  Gain=0.01
  I1 : Gain  Gain=0.1
  Integrator1 : Integrator
  Integrator5 : Integrator
  MATLAB Function : MATLAB Function  TreatAsAtomicUnit=on
  MATLAB Function1 : MATLAB Function  TreatAsAtomicUnit=on
  MATLAB Function19 : MATLAB Function  TreatAsAtomicUnit=on
  P : Gain
  P1 : Gain
  P2 : Gain  Gain=2.26
  Scope1 : Scope  NumInputPorts=2
  Scope{2..5,10,28..29} (7 alike) : Scope
  Sum : Sum  Inputs=|-+-
  Sum1 : Sum  Inputs=|+++
  Sum2 : Sum  Inputs=|++
  Sum3 : Sum  Inputs=|++-
  Sum4 : Sum  Inputs=|+-
  Sum5 : Sum  Inputs=|+++
  Varying Lowpass Filter : cstblocks/Linear Parameter Varying/Varying Lowpass Filter  N=1
  Varying Lowpass Filter1 : cstblocks/Linear Parameter Varying/Varying Lowpass Filter  N=1
  fr2 : Constant  Value=2
  rudder angle : Outport
  rudder angle1 : Outport  Port=2
  wires:
  Varying Lowpass Filter/1 -> MATLAB Function/1(u)
  MATLAB Function/1(y) -> Scope1/1
  Sum1/1 -> Varying Lowpass Filter/1
  I/1 -> Sum1/1
  Sum/1 -> Scope10/1, Derivative/1, Integrator5/1, P/1
  fr2/1 -> Varying Lowpass Filter/2, Varying Lowpass Filter1/2
  D/1 -> Sum1/3
  P/1 -> Sum1/2
  Derivative/1 -> D/1
  Integrator5/1 -> I/1
  MATLAB Function19/2(y1) -> Sum3/2, Gain1/1, Gain12/1, Scope29/1
  MATLAB Function19/1(y) -> Scope28/1
  u/1 -> MATLAB Function19/2(u)
  v/1 -> MATLAB Function19/1(v)
  max rudder angle/1 -> MATLAB Function1/2(max), MATLAB Function/2(max)
  desired heading/1 -> Sum3/1, Sum/2, Scope2/1, Sum2/1
  Sum2/1 -> rudder angle1/1
  Gain1/1 -> Sum2/2
  Sum3/1 -> Scope4/1, P1/1
  P1/1 -> Sum4/1
  r/1 -> Sum4/2
  Sum4/1 -> Scope5/1, Derivative1/1, Integrator1/1, P2/1
  I1/1 -> Sum5/1
  Integrator1/1 -> I1/1
  P2/1 -> Sum5/2
  Derivative1/1 -> D1/1
  D1/1 -> Sum5/3
  MATLAB Function1/1(y) -> rudder angle/1, Scope1/2
  Sum5/1 -> Varying Lowpass Filter1/1
  Varying Lowpass Filter1/1 -> MATLAB Function1/1(u)
  Gain12/1 -> Sum/3
  psi/1 -> Sum3/3, Sum/1

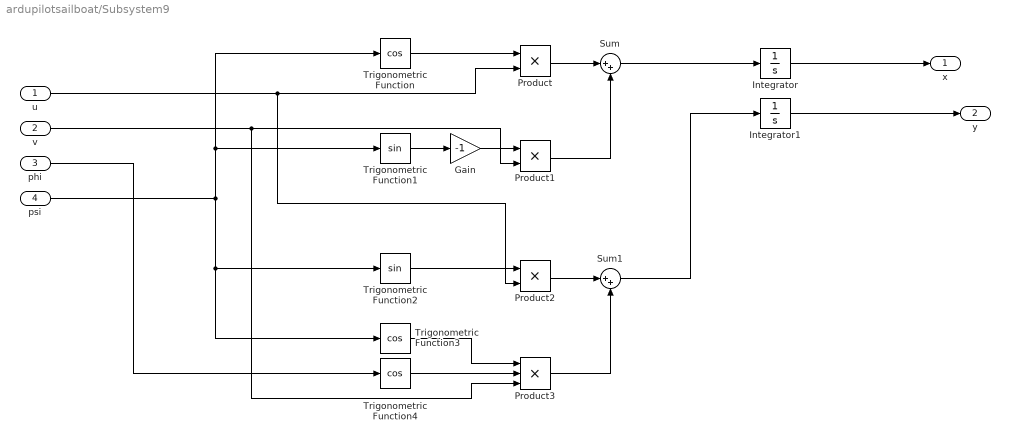
== system ardupilotsailboat/Subsystem9 ==
  u : Inport
  v : Inport  Port=2
  phi : Inport  Port=3
  psi : Inport  Port=4
  Gain : Gain  Gain=-1
  Integrator : Integrator
  Integrator1 : Integrator
  Product : Product
  Product1 : Product
  Product2 : Product
  Product3 : Product  Inputs=3
  Sum : Sum  Inputs=|++
  Sum1 : Sum  Inputs=|++
  Trigonometric Function : Trigonometry  Operator=cos
  Trigonometric Function1 : Trigonometry
  Trigonometric Function2 : Trigonometry
  Trigonometric Function3 : Trigonometry  Operator=cos
  Trigonometric Function4 : Trigonometry  Operator=cos
  x : Outport
  y : Outport  Port=2
  wires:
  Integrator/1 -> x/1
  Integrator1/1 -> y/1
  psi/1 -> Trigonometric Function1/1, Trigonometric Function/1, Trigonometric Function3/1, Trigonometric Function2/1
  Trigonometric Function/1 -> Product/1
  u/1 -> Product/2, Product2/2
  Trigonometric Function1/1 -> Gain/1
  Gain/1 -> Product1/1
  v/1 -> Product1/2, Product3/3
  Product/1 -> Sum/1
  Product1/1 -> Sum/2
  Sum/1 -> Integrator/1
  Product3/1 -> Sum1/2
  Sum1/1 -> Integrator1/1
  Trigonometric Function2/1 -> Product2/1
  Product2/1 -> Sum1/1
  Trigonometric Function3/1 -> Product3/1
  Trigonometric Function4/1 -> Product3/2
  phi/1 -> Trigonometric Function4/1

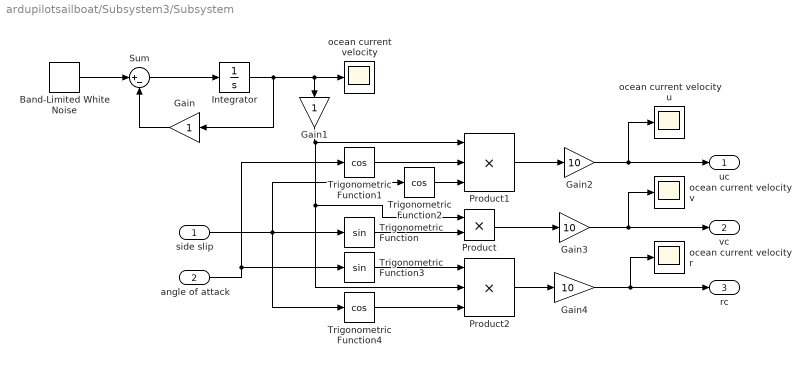
== system ardupilotsailboat/Subsystem3/Subsystem ==
  side slip : Inport
  angle of attack : Inport  Port=2
  Band-Limited White Noise : simulink/Sources/Band-Limited White Noise  Cov=[0.03]  Ts=1  seed=[23341]
  Gain : Gain
  Gain1 : Gain
  Gain2 : Gain  Gain=10
  Gain3 : Gain  Gain=10
  Gain4 : Gain  Gain=10
  Integrator : Integrator
  Product : Product
  Product1 : Product  Inputs=3
  Product2 : Product  Inputs=3
  Sum : Sum  Inputs=|+-
  Trigonometric Function : Trigonometry
  Trigonometric Function1 : Trigonometry  Operator=cos
  Trigonometric Function2 : Trigonometry  Operator=cos
  Trigonometric Function3 : Trigonometry
  Trigonometric Function4 : Trigonometry  Operator=cos
  ocean current velocity : Scope
  ocean current velocity r : Scope
  ocean current velocity u : Scope
  ocean current velocity v : Scope
  uc : Outport
  vc : Outport  Port=2
  rc : Outport  Port=3
  wires:
  Sum/1 -> Integrator/1
  Band-Limited White Noise/1 -> Sum/1
  Integrator/1 -> ocean current velocity/1, Gain1/1, Gain/1
  Gain/1 -> Sum/2
  Trigonometric Function/1 -> Product/2
  side slip/1 -> Trigonometric Function4/1, Trigonometric Function2/1, Trigonometric Function/1
  Product/1 -> Gain3/1
  Trigonometric Function2/1 -> Product1/3
  Trigonometric Function1/1 -> Product1/2
  Product1/1 -> Gain2/1
  Trigonometric Function3/1 -> Product2/1
  Trigonometric Function4/1 -> Product2/3
  angle of attack/1 -> Trigonometric Function3/1, Trigonometric Function1/1
  Product2/1 -> Gain4/1
  Gain1/1 -> Product1/1, Product2/2, Product/1
  Gain2/1 -> ocean current velocity u/1, uc/1
  Gain3/1 -> ocean current velocity v/1, vc/1
  Gain4/1 -> rc/1, ocean current velocity r/1

== matlab function ardupilotsailboat/MATLAB Function3 ==
  data: Xs output; delta_s input; apparent_velocity input; Ys output; Ks output; Ns output; awa output; apparent_wind_angle input; phi input
function [Xs,Ys,Ks,Ns,awa] = sailForce(delta_s,apparent_velocity,apparent_wind_angle,phi)
%Parameters
rho_a = 1.2;
area_sail =0.38;
l1 =0;
l2 = 0;
h1 = 0.6;

% CoE of sail
zs = 0.6;
xs=0;
ys=0;

% Apparent Wind Velocity
awa=apparent_wind_angle;

% Calculate Angle of Attack
alpha = awa-delta_s;


% Calculate Lift and Drag Force
[Cls,Cds] = sailcoef(alpha);
Ls = 0.5*rho_a*area_sail*(apparent_velocity)*Cls;
Ds = 0.5*rho_a*area_sail*(apparent_velocity)*Cds;

% Sail Force components
Xs = (Ls * sin(awa) - Ds * cos(awa));
Ys = (Ls * cos(awa) + Ds * sin(awa))*cos(phi);
Ks =- h1 *(Ls * cos(awa) + Ds * sin(awa));
Ns = (-Xs * l2 * sin(delta_s) + Ys*(l1 - l2*cos(delta_s)));

function [Cls,Cds] = sailcoef(attack)
% generate a lookup table for the lift/drag coefficients for the sail
% and compute Cls/Cds from the lookup table using interpolation.

% lookup table
xdata = linspace(-pi,pi,73); % every 5 degrees
xdata = xdata/pi*180;

% lift curve
yldata = [fliplr([0 0.15 0.32 ...
    0.48 0.7 0.94 1.15 1.3 1.28 1.15 1.1 1.05 1 0.9 0.82 0.72 0.68 0.56 0.48 0.32 0.21 0.08 ...
    -0.06 -0.18 -0.3 -0.4 -0.53 -0.64 -0.72 -0.84 -0.95 -1.04 -1.1 -1.14 -1.08 -0.76 0])*(-1) ...
    [0.15 0.32 ...
    0.48 0.7 0.94 1.15 1.3 1.28 1.15 1.1 1.05 1 0.9 0.82 0.72 0.68 0.56 0.48 0.32 0.21 0.08 ...
    -0.06 -0.18 -0.3 -0.4 -0.53 -0.64 -0.72 -0.84 -0.95 -1.04 -1.1 -1.14 -1.08 -0.76 0]];

% drag curve
yddata = [fliplr([0.1 0.12 0.14 ...
    0.16 0.19 0.26 0.35 0.46 0.54 0.62 0.7 0.78 0.9 0.98 1.04 1.08 1.16 1.2 1.24 1.26 ...
    1.28 1.34 1.36 1.37 1.33 1.31 1.28 1.26 1.25 1.2 1.1 1.04 0.88 0.8 0.64 0.38 0.1])...
    [0.12 0.14 ...
    0.16 0.19 0.26 0.35 0.46 0.54 0.62 0.7 0.78 0.9 0.98 1.04 1.08 1.16 1.2 1.24 1.26 ...
    1.28 1.34 1.36 1.37 1.33 1.31 1.28 1.26 1.25 1.2 1.1 1.04 0.88 0.8 0.64 0.38 0.1]];

% fit the input angle of attack into the interval [-pi,pi]
if attack > pi
    attack = mod(attack+pi,2*pi) - pi;
else
    if attack < -pi
        attack = mod(attack-pi,-2*pi) + pi;
    end
end

% interpolation
attack = attack/pi*180;
Cls = interp1(xdata,yldata,attack,'pchip');
Cds = interp1(xdata,yddata,attack,'pchip');

== matlab function ardupilotsailboat/MATLAB Function4 ==
  data: r input; u input; Xr output; v input; Yr output; Kr output; Nr output; delta_r input; delta_r output; alpha_a output
function [Xr,Yr,Kr,Nr,delta_r,alpha_a] = rudderForce(r,u,v,delta_r)
%Parameters
rudder_width = 4;
rudder_length = 20;
rho_w = 1025;
area = rudder_length * rudder_width * 10^(-4);
velocity = sqrt(v^2+u^2);
l4 = 0.48;
h3 = 0.2;
yr = 0;
xr = -0.5;
zr = 0.2;

% Calculate Angle of Attack
v_aru = -u;
v_arv = -v-r;
alpha_ar = atan2(real(v_arv),real(v_aru));
alpha_a = alpha_ar - delta_r;

% Lift and Drag Coeff
[lc, dc] = ruddercoef(alpha_a);


% Calculate Lift and Drag Force
lift_force = 0.5 * rho_w * area * lc * velocity^2 ;
drag_force = 0.5 * rho_w * area * dc * velocity^2 ;

Xr = (lift_force * sin(alpha_ar) - drag_force * cos(alpha_ar));
Yr = (lift_force * cos(alpha_ar) + drag_force * sin(alpha_ar))*0.1;
Kr =( h3 * ( -lift_force * cos(alpha_ar) - drag_force * sin(alpha_ar)));
Nr = (l4 * (lift_force * cos(alpha_ar) + drag_force * sin(alpha_ar)));


function [Clr,Cdr] = ruddercoef(attack)
% generate a lookup table for the lift/drag coefficients for the sail
% and compute Cls/Cds from the lookup table using interpolation.

% lookup table
xdata = linspace(-pi,pi,73); % every 5 degrees
xdata = xdata/pi*180;

% lift curve
yl = fliplr([0 0.42 0.73 ...
    0.95 1.1 1.165 1.18 1.155 1.12 1.065 1 0.92 0.83 0.72 0.62 0.48 0.33 0.16])*(-1);
yldata = [fliplr([0 0.42 0.73 ...
    0.95 1.1 1.165 1.18 1.155 1.12 1.065 1 0.92 0.83 0.72 0.62 0.48 0.33 0.16 0 yl])*(-1) ...
    [0.42 0.73 ...
    0.95 1.1 1.165 1.18 1.155 1.12 1.065 1 0.92 0.83 0.72 0.62 0.48 0.33 0.16 0 yl]];

% drag curve
yd = fliplr([0 0.03 0.06 ...
    0.1 0.17 0.3 0.48 0.74 0.98 1.18 1.34 1.5 1.65 1.76 1.89 1.97 2.01 2.05]);
yddata = [fliplr([0 0.03 0.06 ...
    0.1 0.17 0.3 0.48 0.74 0.98 1.18 1.34 1.5 1.65 1.76 1.89 1.97 2.01 2.05 2.08 yd])...
    [0.03 0.06 ...
    0.1 0.17 0.3 0.48 0.74 0.98 1.18 1.34 1.5 1.65 1.76 1.89 1.97 2.01 2.05 2.08 yd]];

% fit the input angle of attack into the interval [-pi,pi]
if attack > pi
    attack = mod(attack+pi,2*pi) - pi;
else
    if attack < -pi
        attack = mod(attack-pi,-2*pi) + pi;
    end
end

% interpolation
attack = attack/pi*180;
Clr = interp1(xdata,yldata,attack,'pchip');
Cdr = interp1(xdata,yddata,attack,'pchip');

== matlab function ardupilotsailboat/MATLAB Function5 ==
  data: r input; u input; Xk output; v input; Yk output; Kk output; Nk output; phi input
function [Xk,Yk,Kk,Nk] = keelForce(r,u,v,phi)
%Parameters
keel_width = 8;
keel_length = 45;
rho_w = 1025;
area = keel_width * keel_length * 10^(-4);
velocity = sqrt(v^2+u^2);
l3 = 0.1;
h2 = 0.275;
yk=0;
xk=0.1;
zk=0.25;

% Calculate Angle of Attack
v_aku = -u + r*yk;
v_akv = -v - r*xk + 0*zk;
alpha_ak = atan2(real(v_akv),real(-v_aku));
alpha = alpha_ak;

% Lift and Drag Coeff
[lc, dc] = keelcoef(alpha);

% Calculate Lift and Drag Force
lift_force = 0.5 * rho_w * area * lc * (v_aku^2+v_akv^2);
drag_force = 0.5 * rho_w * area * dc * (v_aku^2+v_akv^2);

Xk = (-lift_force * sin(alpha_ak) + drag_force * cos(alpha_ak));
Yk = (-lift_force * cos(alpha_ak) - drag_force * sin(alpha_ak))*cos(phi);
Kk = -(-lift_force*cos(alpha_ak)-drag_force*sin(alpha_ak))*zk;
Nk = -(lift_force*cos(alpha_ak)+drag_force*sin(alpha_ak))*xk;




%------------------------------------------------------------------------------------------------------------------------------
function [Clk,Cdk] = keelcoef(attack)
% generate a lookup table for the lift/drag coefficients for the sail
% and compute Cls/Cds from the lookup table using interpolation.

% lookup table
xdata = linspace(-pi,pi,73); % every 5 degrees
xdata = xdata/pi*180;

% lift curve
yl = fliplr([0 0.425 0.74 ...
    0.94 1.1 1.17 1.19 1.16 1.12 1.07 0.99 0.92 0.84 0.74 0.63 0.49 0.345 0.185])*(-1);
yldata = [fliplr([0 0.425 0.74 ...
    0.94 1.1 1.17 1.19 1.16 1.12 1.07 0.99 0.92 0.84 0.74 0.63 0.49 0.345 0.185 0 yl])*(-1) ...
    [0.425 0.74 ...
    0.94 1.1 1.17 1.19 1.16 1.12 1.07 0.99 0.92 0.84 0.74 0.63 0.49 0.345 0.185 0 yl]];

% drag curve
yd = fliplr([0 0.04 0.07 ...
    0.1 0.17 0.3 0.49 0.76 0.98 1.19 1.34 1.5 1.65 1.77 1.88 1.96 2.01 2.05]);
yddata = [fliplr([0 0.04 0.07 ...
    0.1 0.17 0.3 0.49 0.76 0.98 1.19 1.34 1.5 1.65 1.77 1.88 1.96 2.01 2.05 2.09 yd])...
    [0.04 0.07 ...
    0.1 0.17 0.3 0.49 0.76 0.98 1.19 1.34 1.5 1.65 1.77 1.88 1.96 2.01 2.05 2.09 yd]];

% fit the input angle of attack into the interval [-pi,pi]
if attack > pi
    attack = mod(attack+pi,2*pi) - pi;
else
    if attack < -pi
        attack = mod(attack-pi,-2*pi) + pi;
    end
end

% interpolation
attack = attack/pi*180;
Clk = interp1(xdata,yldata,attack,'pchip');
Cdk = interp1(xdata,yddata,attack,'pchip');


%------------------------------------------------------------------------------------------------------------------------------
function F = resistancehull(alpha_a)

xdata = linspace(0,6,13); % every 0.5m/s
ydata = [0 0.15 0.35 0.5 0.675 0.825 1.175 1.4 2 4.85 9.85 18.46 27.5]*1000;

% interpolation
if alpha_a <= 6
    F = interp1(xdata,ydata,alpha_a,'pchip');
else
    F = interp1(xdata,ydata,alpha_a,'pchip','extrap');
end
